simulink model "PneumaticDigitalTwin"  (R2025b)
settings: Solver=ode4  StartTime=0.0  StopTime=20  FixedStep=0.02  RelTol=1e-3
undefined symbols (not defined in the file): faultId, Ts
settings Model: Creator=merie  LastModifiedBy=merie

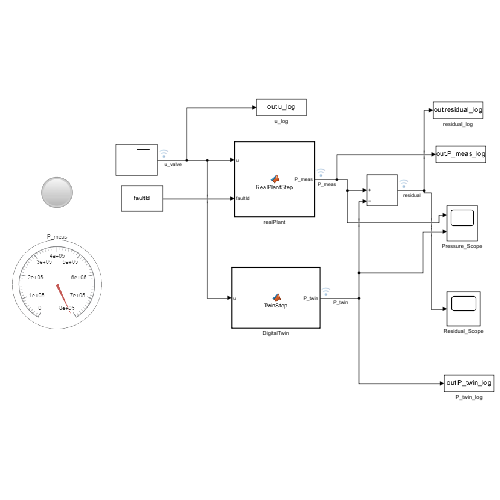
[thumbnail: Simulink's stored preview of the top-level diagram]
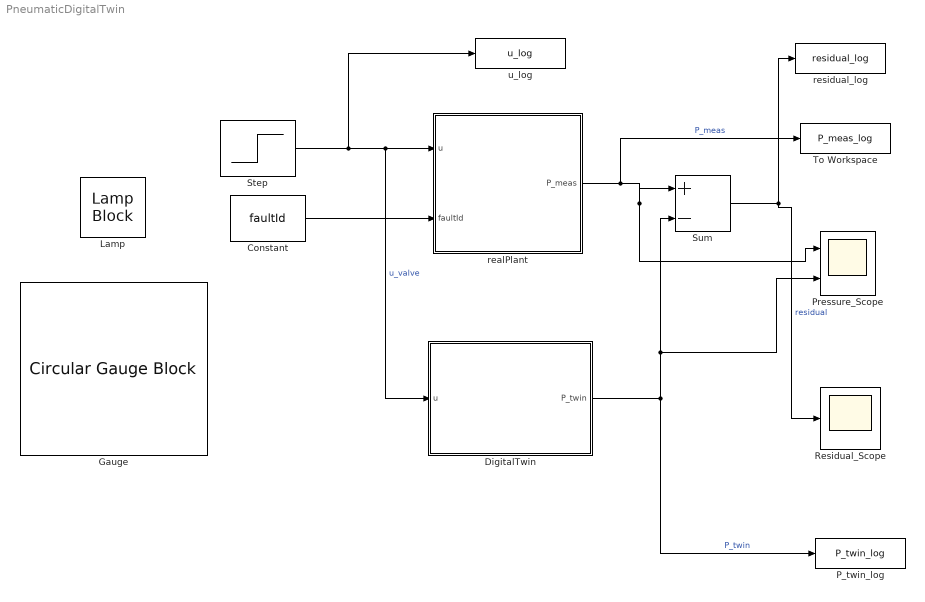
== system PneumaticDigitalTwin ==
  Constant : Constant  Value=faultId  OutDataTypeStr=uint8  LockScale=on
  DigitalTwin : MATLAB Function  TreatAsAtomicUnit=on
  Gauge : CircularGaugeBlock  ScaleMax=800000  TickInterval=100000  FontColor=[0.0, 0.0, 0.0]
  Lamp : LampBlock  LabelPosition=Hide  DefaultColor=[192.0, 192.0, 192.0]
  P_twin_log : ToWorkspace  VariableName=P_twin_log  SampleTime=-1
  Pressure_Scope : Scope  NumInputPorts=2
      settings: ActiveDisplayYMinimum=-1.4791229280971675E+6  ActiveDisplayYMaximum=1.3967374769788576E+7  DataLoggingVariableName=pressure_data
  Residual_Scope : Scope
      settings: ActiveDisplayYMinimum=-35998.958048376757  ActiveDisplayYMaximum=-34001.019558895554
  Step : Step  Time=5  Before=0.3  After=0.8  SampleTime=Ts
  Sum : Sum  Inputs=|+-
  To Workspace : ToWorkspace  VariableName=P_meas_log  SampleTime=-1
  realPlant : MATLAB Function  TreatAsAtomicUnit=on
  residual_log : ToWorkspace  VariableName=residual_log  SampleTime=-1
  u_log : ToWorkspace  VariableName=u_log  SampleTime=-1
  wires:
  Step/1 -> u_log/1, DigitalTwin/1(u), realPlant/1(u)  "u_valve"
  Constant/1 -> realPlant/2(faultId)
  realPlant/1(P_meas) -> To Workspace/1, Pressure_Scope/1, Sum/1  "P_meas"
  DigitalTwin/1(P_twin) -> P_twin_log/1, Pressure_Scope/2, Sum/2  "P_twin"
  Sum/1 -> residual_log/1, Residual_Scope/1  "residual"

== matlab function PneumaticDigitalTwin/realPlant ==
  data: u input; P_meas output; faultId input
function P_meas = RealPlantStep(u, faultId)
%#codegen
% Real pneumatic plant with fault injection
% Inputs:
%   u       - valve command [0, 1]
%   faultId - fault type: 0=normal, 1-7=various faults
% Output:
%   P_meas  - measured pressure [Pa]

    persistent P
    if isempty(P)
        P = 1.01325e5;  % Initial atmospheric pressure
    end
    
    % ===== PHYSICAL PARAMETERS =====
    Ts = 0.02;                  % Sample time (must match Simulink)
    Ps = 7e5;                   % Supply pressure (7 bar gauge)
    Patm = 1.01325e5;           % Atmospheric pressure
    C = 1.5e-9;                 % Volume capacitance
    R_in_nominal = 5e5;         % Nominal inlet resistance
    R_leak_nominal = 3e6;       % Nominal leak resistance
    
    % ===== SENSOR PARAMETERS =====
    sensorNoise = 800;          % Gaussian noise std dev [Pa]
    sensorBias_pos = 4e4;       % Positive bias [Pa]
    sensorBias_neg = -3.5e4;    % Negative bias [Pa]
    
    % ===== FAULT CONFIGURATION =====
    leakFactor = 1.0;           % 1.0 = no leak, <1.0 = more leak
    valveStuck = false;
    valveStuckValue = 0.5;
    sensorBias = 0.0;
    
    % Map faultId to specific fault parameters
    if faultId == uint8(0)
        % Normal operation - no changes needed
        
    elseif faultId == uint8(1)
        % Small leak
        leakFactor = 0.40;
        
    elseif faultId == uint8(2)
        % Large leak
        leakFactor = 0.12;
        
    elseif faultId == uint8(3)
        % Critical leak
        leakFactor = 0.05;
        
    elseif faultId == uint8(4)
        % Valve stuck at half open
        valveStuck = true;
        valveStuckValue = 0.5;
        
    elseif faultId == uint8(5)
        % Valve stuck closed
        valveStuck = true;
        valveStuckValue = 0.05;
        
    elseif faultId == uint8(6)
        % Positive sensor bias
        sensorBias = sensorBias_pos;
        
    elseif faultId == uint8(7)
        % Negative sensor bias
        sensorBias = sensorBias_neg;
    end
    
    % ===== APPLY VALVE FAULT =====
    if valveStuck
        u_eff = valveStuckValue;
    else
        u_eff = u;
    end
    
    % Clamp valve command
    u_eff = max(min(u_eff, 1.0), 0.05);
    
    % ===== PHYSICS SIMULATION =====
    R_leak_real = R_leak_nominal * leakFactor;
    Rin = R_in_nominal / u_eff;
    
    % First-order dynamics: dP/dt = (Ps - P)/(C*Rin) - P/(C*R_leak)
    dPdt = (Ps - P) / (C * Rin) - P / (C * R_leak_real);
    
    % Euler integration
    P = P + Ts * dPdt;
    
    % Physical constraint: pressure cannot go below atmospheric
    P = max(P, Patm);
    
    % ===== SENSOR MEASUREMENT =====
    % Add Gaussian noise
    noise = sensorNoise * (2*rand() - 1);  % Uniform approximation for codegen
    
    % Final measurement
    P_meas = P + sensorBias + noise;
    
    % Ensure measurement is physical
    P_meas = max(P_meas, 0);
end

== matlab function PneumaticDigitalTwin/DigitalTwin ==
  data: u input; P_twin output
function P_twin = TwinStep(u)
%#codegen
% Ideal digital twin - no faults, nominal parameters
% Input:
%   u      - valve command [0, 1]
% Output:
%   P_twin - twin pressure estimate [Pa]

    persistent P
    if isempty(P)
        P = 1.01325e5;  % Initial atmospheric pressure
    end
    
    % ===== NOMINAL PARAMETERS (NO FAULTS) =====
    Ts = 0.02;                  % Sample time
    Ps = 7e5;                   % Supply pressure
    Patm = 1.01325e5;           % Atmospheric pressure
    C = 1.5e-9;                 % Volume capacitance
    R_in_nominal = 5e5;         % Inlet resistance
    R_leak_nominal = 3e6;       % Nominal leak resistance (no fault)
    
    % Clamp valve command
    u_eff = max(min(u, 1.0), 0.05);
    
    % ===== PHYSICS SIMULATION =====
    Rin = R_in_nominal / u_eff;
    
    % Dynamics
    dPdt = (Ps - P) / (C * Rin) - P / (C * R_leak_nominal);
    
    % Euler integration
    P = P + Ts * dPdt;
    
    % Physical constraint
    P = max(P, Patm);
    
    % Output (no sensor noise in twin)
    P_twin = P;
end
